simulink model "pmramp"  (R2018a)
settings: Solver=VariableStepAuto  StartTime=0.0  StopTime=1  RelTol=1e-3
libraries: simulink x1
settings Model: Creator=pc  LastModifiedBy=pc

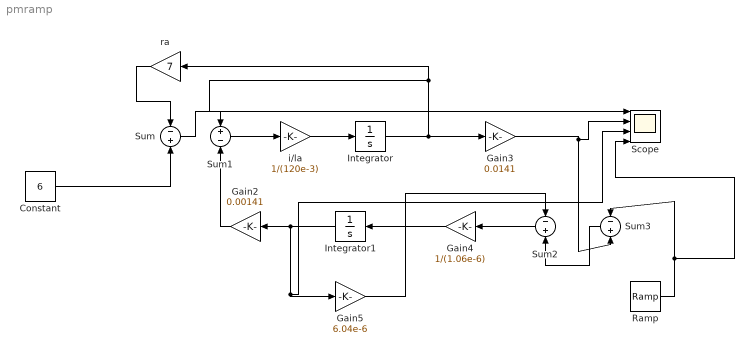
== system pmramp ==
  Constant : Constant  Value=6
  Gain2 : Gain  Gain=0.00141
  Gain3 : Gain  Gain=0.0141
  Gain4 : Gain  Gain=1/(1.06e-6)
  Gain5 : Gain  Gain=6.04e-6
  Integrator : Integrator
  Integrator1 : Integrator
  Ramp : simulink/Sources/Ramp  slope=0.025  start=0.5  InitialOutput=0
  Scope : Scope  NumInputPorts=4
  Sum : Sum  Inputs=-+
  Sum1 : Sum  Inputs=+-
  Sum2 : Sum  Inputs=-+
  Sum3 : Sum  Inputs=-+
  i/la : Gain  Gain=1/(120e-3)
  ra : Gain  Gain=7
  wires:
  Ramp/1 -> Scope/4, Sum3/1
  Constant/1 -> Sum/2
  Sum2/1 -> Gain4/1
  Integrator1/1 -> Scope/3, Gain5/1, Gain2/1
  Gain3/1 -> Scope/2, Sum3/2
  i/la/1 -> Integrator/1
  Gain2/1 -> Sum1/2
  Integrator/1 -> Scope/1, ra/1, Gain3/1
  Sum3/1 -> Sum2/2
  Gain4/1 -> Integrator1/1
  Gain5/1 -> Sum2/1
  ra/1 -> Sum/1
  Sum1/1 -> i/la/1
  Sum/1 -> Sum1/1
